simulink model "PIDLoopTest_Multiple"  (R2014a)
settings: Solver=ode3  SolverMode=SingleTasking  StartTime=0.0  StopTime=inf  RelTol=1e-3
libraries: arduinolib x13, simulink x12
settings Model: ExtModeTrigDuration=2  Creator=paddockt  LastModifiedBy=paddockt
settings OptimizationCC: OptimizeModelRefInitCode=on  LifeSpan=1
settings DebuggingCC: UnderspecifiedInitializationDetection=Classic  SolverPrmCheckMsg=none
settings HardwareCC: ProdBitPerInt=16  ProdBitPerPointer=8  ProdIntDivRoundTo=Zero  ProdEndianess=LittleEndian  ProdWordSize=8  ProdHWDeviceType=Atmel->AVR
settings RTWCC: SystemTargetFile=realtime.tlc  GenerateMakefile=off  TemplateMakefile=realtime.tmf  Description=Run on Target Hardware  RTWVerbose=off  ProcessScript=realtime_make_rtw_hook
settings STFCustomTargetCC: TargetLibSuffix=.a  GenerateSampleERTMain=on  ConcurrentExecutionCompliant=off  GeneratePreprocessorConditionals=Use local settings  ERTCustomFileBanners=on  SupportNonInlinedSFcns=off  SupportVariableSizeSignals=on  MATLABClassNameForMDSCustomization=Simulink.SoftwareTarget.ERTCustomization  GRTInterface=off  SystemTargetFile=realtime.tlc
settings ERTTargetCC: CombineOutputUpdateFcns=off  SupportContinuousTime=on  SupportVariableSizeSignals=on  ExtModeMexArgs='192.168.1.20' 1 17725  ERTSrcFileBannerTemplate=realtime_code_template.cgt  ERTHdrFileBannerTemplate=realtime_code_template.cgt  ERTDataSrcFileTemplate=realtime_code_template.cgt  ERTDataHdrFileTemplate=realtime_code_template.cgt  ERTCustomFileTemplate=realtime_file_process.tlc

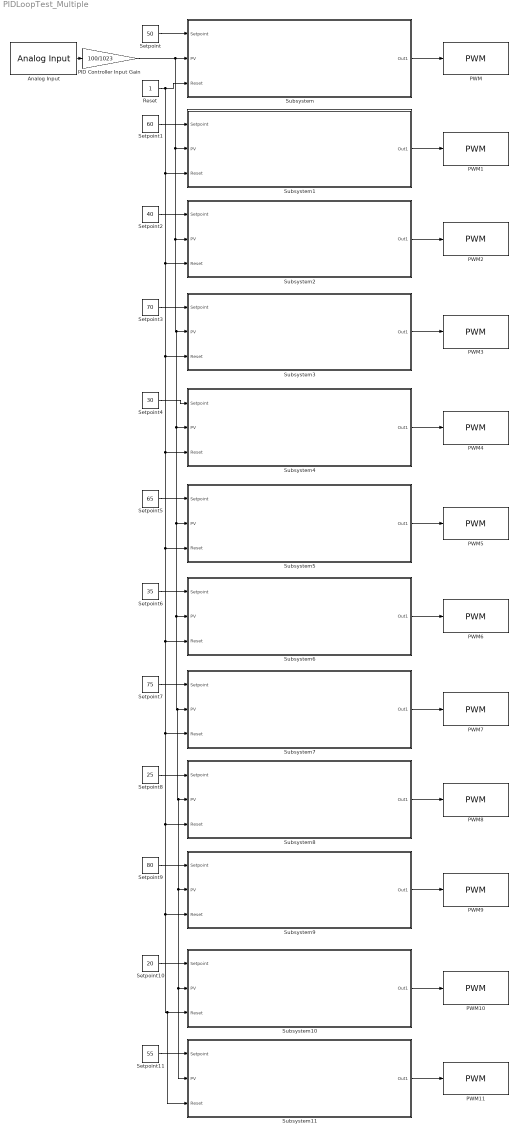
== system PIDLoopTest_Multiple ==
  Analog Input : arduinolib/Analog Input  pinNumber=0  sampleTime=1
  PID Controller Input Gain : Gain  Gain=100/1023
  PWM : arduinolib/PWM  pinNumber=13
  PWM1 : arduinolib/PWM  pinNumber=12
  PWM10 : arduinolib/PWM  pinNumber=3
  PWM11 : arduinolib/PWM  pinNumber=2
  PWM2 : arduinolib/PWM  pinNumber=11
  PWM3 : arduinolib/PWM  pinNumber=10
  PWM4 : arduinolib/PWM  pinNumber=9
  PWM5 : arduinolib/PWM  pinNumber=8
  PWM6 : arduinolib/PWM  pinNumber=7
  PWM7 : arduinolib/PWM  pinNumber=6
  PWM8 : arduinolib/PWM  pinNumber=5
  PWM9 : arduinolib/PWM  pinNumber=4
  Reset : Constant
  Setpoint : Constant  Value=50
  Setpoint1 : Constant  Value=60
  Setpoint10 : Constant  Value=20
  Setpoint11 : Constant  Value=55
  Setpoint2 : Constant  Value=40
  Setpoint3 : Constant  Value=70
  Setpoint4 : Constant  Value=30
  Setpoint5 : Constant  Value=65
  Setpoint6 : Constant  Value=35
  Setpoint7 : Constant  Value=75
  Setpoint8 : Constant  Value=25
  Setpoint9 : Constant  Value=80
  Subsystem : Subsystem
  Subsystem1 : Subsystem
  Subsystem10 : Subsystem
  Subsystem11 : Subsystem
  Subsystem2 : Subsystem
  Subsystem3 : Subsystem
  Subsystem4 : Subsystem
  Subsystem5 : Subsystem
  Subsystem6 : Subsystem
  Subsystem7 : Subsystem
  Subsystem8 : Subsystem
  Subsystem9 : Subsystem
  wires:
  Analog Input/1 -> PID Controller Input Gain/1
  PID Controller Input Gain/1 -> Subsystem11/2(PV), Subsystem10/2(PV), Subsystem9/2(PV), Subsystem8/2(PV), Subsystem7/2(PV), Subsystem6/2(PV), Subsystem5/2(PV), Subsystem4/2(PV), Subsystem3/2(PV), Subsystem2/2(PV), Subsystem1/2(PV), Subsystem/2(PV)
  Setpoint/1 -> Subsystem/1(Setpoint)
  Reset/1 -> Subsystem11/3(Reset), Subsystem10/3(Reset), Subsystem9/3(Reset), Subsystem8/3(Reset), Subsystem7/3(Reset), Subsystem6/3(Reset), Subsystem5/3(Reset), Subsystem4/3(Reset), Subsystem3/3(Reset), Subsystem2/3(Reset), Subsystem1/3(Reset), Subsystem/3(Reset)
  Subsystem/1(Out1) -> PWM/1
  Subsystem1/1(Out1) -> PWM1/1
  Subsystem2/1(Out1) -> PWM2/1
  Subsystem3/1(Out1) -> PWM3/1
  Subsystem4/1(Out1) -> PWM4/1
  Subsystem5/1(Out1) -> PWM5/1
  Subsystem6/1(Out1) -> PWM6/1
  Subsystem7/1(Out1) -> PWM7/1
  Subsystem8/1(Out1) -> PWM8/1
  Subsystem9/1(Out1) -> PWM9/1
  Subsystem10/1(Out1) -> PWM10/1
  Subsystem11/1(Out1) -> PWM11/1
  Setpoint1/1 -> Subsystem1/1(Setpoint)
  Setpoint2/1 -> Subsystem2/1(Setpoint)
  Setpoint3/1 -> Subsystem3/1(Setpoint)
  Setpoint4/1 -> Subsystem4/1(Setpoint)
  Setpoint5/1 -> Subsystem5/1(Setpoint)
  Setpoint6/1 -> Subsystem6/1(Setpoint)
  Setpoint7/1 -> Subsystem7/1(Setpoint)
  Setpoint8/1 -> Subsystem8/1(Setpoint)
  Setpoint9/1 -> Subsystem9/1(Setpoint)
  Setpoint10/1 -> Subsystem10/1(Setpoint)
  Setpoint11/1 -> Subsystem11/1(Setpoint)

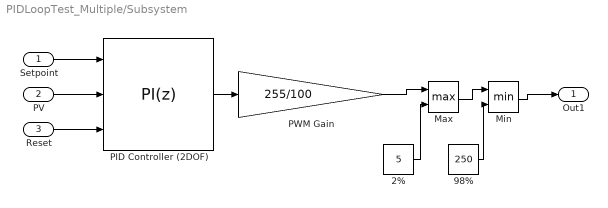
== system PIDLoopTest_Multiple/Subsystem ==
  Setpoint : Inport
  PV : Inport  Port=2
  Reset : Inport  Port=3
  2% : Constant  Value=5
  98% : Constant  Value=250
  Max : MinMax  Function=max  Inputs=2
  Min : MinMax  Inputs=2
  PID Controller (2DOF) : simulink/Continuous/PID Controller (2DOF)  Controller=PI  TimeDomain=Discrete-time  SampleTime=1  IntegratorMethod=Forward Euler  FilterMethod=Forward Euler  Form=Parallel  P=1  I=1  D=0  N=100  b=1  c=1  InitialConditionSource=internal  InitialConditionForIntegrator=0  InitialConditionForFilter=0  ExternalReset=falling  LimitOutput=on  UpperSaturationLimit=100  LowerSaturationLimit=0  LinearizeAsGain=on  AntiWindupMode=none  Kb=1  TrackingMode=off  Kt=1  PParamMin=[]  PParamMax=[]  IParamMin=[]  IParamMax=[]  DParamMin=[]  DParamMax=[]  NParamMin=[]  NParamMax=[]  bParamMin=[]  bParamMax=[]  cParamMin=[]  cParamMax=[]  KbParamMin=[]  KbParamMax=[]  KtParamMin=[]  KtParamMax=[]  POutMin=[]  POutMax=[]  IOutMin=[]  IOutMax=[]  DOutMin=[]  DOutMax=[]  NOutMin=[]  NOutMax=[]  bOutMin=[]  bOutMax=[]  cOutMin=[]  cOutMax=[]  KbOutMin=[]  KbOutMax=[]  KtOutMin=[]  KtOutMax=[]  IntegratorOutMin=[]  IntegratorOutMax=[]  FilterOutMin=[]  FilterOutMax=[]  SumOutMin=[]  SumOutMax=[]  Sum1OutMin=[]  Sum1OutMax=[]  Sum2OutMin=[]  Sum2OutMax=[]  Sum3OutMin=[]  Sum3OutMax=[]  SumI1OutMin=[]  SumI1OutMax=[]  SumI2OutMin=[]  SumI2OutMax=[]  SumI3OutMin=[]  SumI3OutMax=[]  SumDOutMin=[]  SumDOutMax=[]  SaturationOutMin=[]  SaturationOutMax=[]  IntegratorContinuousStateAttributes=''  IntegratorStateMustResolveToSignalObject=off  IntegratorRTWStateStorageClass=Auto  FilterContinuousStateAttributes=''  FilterStateMustResolveToSignalObject=off  FilterRTWStateStorageClass=Auto
  PWM Gain : Gain  Gain=255/100
  Out1 : Outport
  wires:
  PID Controller (2DOF)/1 -> PWM Gain/1
  Setpoint/1 -> PID Controller (2DOF)/1
  PWM Gain/1 -> Max/1
  Reset/1 -> PID Controller (2DOF)/3
  PV/1 -> PID Controller (2DOF)/2
  Min/1 -> Out1/1
  Max/1 -> Min/1
  98%/1 -> Min/2
  2%/1 -> Max/2

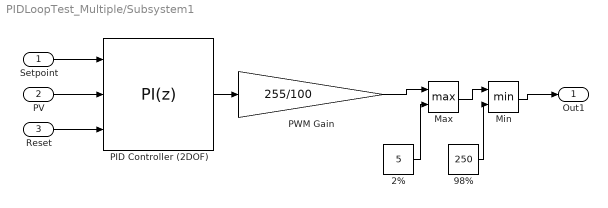
== system PIDLoopTest_Multiple/Subsystem1 ==
  Setpoint : Inport
  PV : Inport  Port=2
  Reset : Inport  Port=3
  2% : Constant  Value=5
  98% : Constant  Value=250
  Max : MinMax  Function=max  Inputs=2
  Min : MinMax  Inputs=2
  PID Controller (2DOF) : simulink/Continuous/PID Controller (2DOF)  Controller=PI  TimeDomain=Discrete-time  SampleTime=1  IntegratorMethod=Forward Euler  FilterMethod=Forward Euler  Form=Parallel  P=1  I=1  D=0  N=100  b=1  c=1  InitialConditionSource=internal  InitialConditionForIntegrator=0  InitialConditionForFilter=0  ExternalReset=falling  LimitOutput=on  UpperSaturationLimit=100  LowerSaturationLimit=0  LinearizeAsGain=on  AntiWindupMode=none  Kb=1  TrackingMode=off  Kt=1  PParamMin=[]  PParamMax=[]  IParamMin=[]  IParamMax=[]  DParamMin=[]  DParamMax=[]  NParamMin=[]  NParamMax=[]  bParamMin=[]  bParamMax=[]  cParamMin=[]  cParamMax=[]  KbParamMin=[]  KbParamMax=[]  KtParamMin=[]  KtParamMax=[]  POutMin=[]  POutMax=[]  IOutMin=[]  IOutMax=[]  DOutMin=[]  DOutMax=[]  NOutMin=[]  NOutMax=[]  bOutMin=[]  bOutMax=[]  cOutMin=[]  cOutMax=[]  KbOutMin=[]  KbOutMax=[]  KtOutMin=[]  KtOutMax=[]  IntegratorOutMin=[]  IntegratorOutMax=[]  FilterOutMin=[]  FilterOutMax=[]  SumOutMin=[]  SumOutMax=[]  Sum1OutMin=[]  Sum1OutMax=[]  Sum2OutMin=[]  Sum2OutMax=[]  Sum3OutMin=[]  Sum3OutMax=[]  SumI1OutMin=[]  SumI1OutMax=[]  SumI2OutMin=[]  SumI2OutMax=[]  SumI3OutMin=[]  SumI3OutMax=[]  SumDOutMin=[]  SumDOutMax=[]  SaturationOutMin=[]  SaturationOutMax=[]  IntegratorContinuousStateAttributes=''  IntegratorStateMustResolveToSignalObject=off  IntegratorRTWStateStorageClass=Auto  FilterContinuousStateAttributes=''  FilterStateMustResolveToSignalObject=off  FilterRTWStateStorageClass=Auto
  PWM Gain : Gain  Gain=255/100
  Out1 : Outport
  wires:
  2%/1 -> Max/2
  98%/1 -> Min/2
  Max/1 -> Min/1
  Min/1 -> Out1/1
  PV/1 -> PID Controller (2DOF)/2
  Reset/1 -> PID Controller (2DOF)/3
  PWM Gain/1 -> Max/1
  Setpoint/1 -> PID Controller (2DOF)/1
  PID Controller (2DOF)/1 -> PWM Gain/1

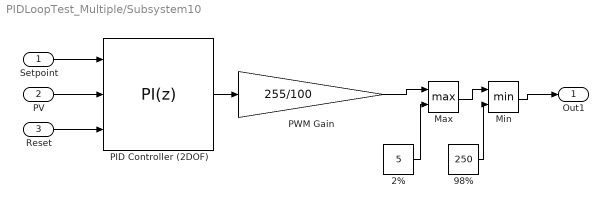
== system PIDLoopTest_Multiple/Subsystem10 ==
  Setpoint : Inport
  PV : Inport  Port=2
  Reset : Inport  Port=3
  2% : Constant  Value=5
  98% : Constant  Value=250
  Max : MinMax  Function=max  Inputs=2
  Min : MinMax  Inputs=2
  PID Controller (2DOF) : simulink/Continuous/PID Controller (2DOF)  Controller=PI  TimeDomain=Discrete-time  SampleTime=1  IntegratorMethod=Forward Euler  FilterMethod=Forward Euler  Form=Parallel  P=1  I=1  D=0  N=100  b=1  c=1  InitialConditionSource=internal  InitialConditionForIntegrator=0  InitialConditionForFilter=0  ExternalReset=falling  LimitOutput=on  UpperSaturationLimit=100  LowerSaturationLimit=0  LinearizeAsGain=on  AntiWindupMode=none  Kb=1  TrackingMode=off  Kt=1  PParamMin=[]  PParamMax=[]  IParamMin=[]  IParamMax=[]  DParamMin=[]  DParamMax=[]  NParamMin=[]  NParamMax=[]  bParamMin=[]  bParamMax=[]  cParamMin=[]  cParamMax=[]  KbParamMin=[]  KbParamMax=[]  KtParamMin=[]  KtParamMax=[]  POutMin=[]  POutMax=[]  IOutMin=[]  IOutMax=[]  DOutMin=[]  DOutMax=[]  NOutMin=[]  NOutMax=[]  bOutMin=[]  bOutMax=[]  cOutMin=[]  cOutMax=[]  KbOutMin=[]  KbOutMax=[]  KtOutMin=[]  KtOutMax=[]  IntegratorOutMin=[]  IntegratorOutMax=[]  FilterOutMin=[]  FilterOutMax=[]  SumOutMin=[]  SumOutMax=[]  Sum1OutMin=[]  Sum1OutMax=[]  Sum2OutMin=[]  Sum2OutMax=[]  Sum3OutMin=[]  Sum3OutMax=[]  SumI1OutMin=[]  SumI1OutMax=[]  SumI2OutMin=[]  SumI2OutMax=[]  SumI3OutMin=[]  SumI3OutMax=[]  SumDOutMin=[]  SumDOutMax=[]  SaturationOutMin=[]  SaturationOutMax=[]  IntegratorContinuousStateAttributes=''  IntegratorStateMustResolveToSignalObject=off  IntegratorRTWStateStorageClass=Auto  FilterContinuousStateAttributes=''  FilterStateMustResolveToSignalObject=off  FilterRTWStateStorageClass=Auto
  PWM Gain : Gain  Gain=255/100
  Out1 : Outport
  wires:
  2%/1 -> Max/2
  98%/1 -> Min/2
  Max/1 -> Min/1
  Min/1 -> Out1/1
  PV/1 -> PID Controller (2DOF)/2
  Reset/1 -> PID Controller (2DOF)/3
  PWM Gain/1 -> Max/1
  Setpoint/1 -> PID Controller (2DOF)/1
  PID Controller (2DOF)/1 -> PWM Gain/1

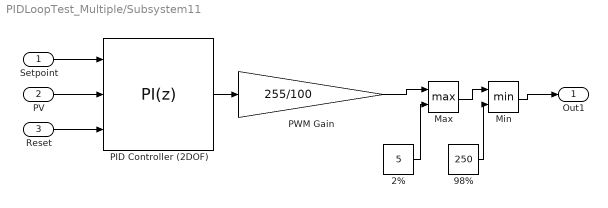
== system PIDLoopTest_Multiple/Subsystem11 ==
  Setpoint : Inport
  PV : Inport  Port=2
  Reset : Inport  Port=3
  2% : Constant  Value=5
  98% : Constant  Value=250
  Max : MinMax  Function=max  Inputs=2
  Min : MinMax  Inputs=2
  PID Controller (2DOF) : simulink/Continuous/PID Controller (2DOF)  Controller=PI  TimeDomain=Discrete-time  SampleTime=1  IntegratorMethod=Forward Euler  FilterMethod=Forward Euler  Form=Parallel  P=1  I=1  D=0  N=100  b=1  c=1  InitialConditionSource=internal  InitialConditionForIntegrator=0  InitialConditionForFilter=0  ExternalReset=falling  LimitOutput=on  UpperSaturationLimit=100  LowerSaturationLimit=0  LinearizeAsGain=on  AntiWindupMode=none  Kb=1  TrackingMode=off  Kt=1  PParamMin=[]  PParamMax=[]  IParamMin=[]  IParamMax=[]  DParamMin=[]  DParamMax=[]  NParamMin=[]  NParamMax=[]  bParamMin=[]  bParamMax=[]  cParamMin=[]  cParamMax=[]  KbParamMin=[]  KbParamMax=[]  KtParamMin=[]  KtParamMax=[]  POutMin=[]  POutMax=[]  IOutMin=[]  IOutMax=[]  DOutMin=[]  DOutMax=[]  NOutMin=[]  NOutMax=[]  bOutMin=[]  bOutMax=[]  cOutMin=[]  cOutMax=[]  KbOutMin=[]  KbOutMax=[]  KtOutMin=[]  KtOutMax=[]  IntegratorOutMin=[]  IntegratorOutMax=[]  FilterOutMin=[]  FilterOutMax=[]  SumOutMin=[]  SumOutMax=[]  Sum1OutMin=[]  Sum1OutMax=[]  Sum2OutMin=[]  Sum2OutMax=[]  Sum3OutMin=[]  Sum3OutMax=[]  SumI1OutMin=[]  SumI1OutMax=[]  SumI2OutMin=[]  SumI2OutMax=[]  SumI3OutMin=[]  SumI3OutMax=[]  SumDOutMin=[]  SumDOutMax=[]  SaturationOutMin=[]  SaturationOutMax=[]  IntegratorContinuousStateAttributes=''  IntegratorStateMustResolveToSignalObject=off  IntegratorRTWStateStorageClass=Auto  FilterContinuousStateAttributes=''  FilterStateMustResolveToSignalObject=off  FilterRTWStateStorageClass=Auto
  PWM Gain : Gain  Gain=255/100
  Out1 : Outport
  wires:
  PID Controller (2DOF)/1 -> PWM Gain/1
  Setpoint/1 -> PID Controller (2DOF)/1
  PWM Gain/1 -> Max/1
  Reset/1 -> PID Controller (2DOF)/3
  PV/1 -> PID Controller (2DOF)/2
  Min/1 -> Out1/1
  Max/1 -> Min/1
  98%/1 -> Min/2
  2%/1 -> Max/2

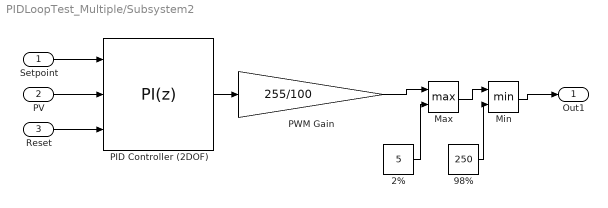
== system PIDLoopTest_Multiple/Subsystem2 ==
  Setpoint : Inport
  PV : Inport  Port=2
  Reset : Inport  Port=3
  2% : Constant  Value=5
  98% : Constant  Value=250
  Max : MinMax  Function=max  Inputs=2
  Min : MinMax  Inputs=2
  PID Controller (2DOF) : simulink/Continuous/PID Controller (2DOF)  Controller=PI  TimeDomain=Discrete-time  SampleTime=1  IntegratorMethod=Forward Euler  FilterMethod=Forward Euler  Form=Parallel  P=1  I=1  D=0  N=100  b=1  c=1  InitialConditionSource=internal  InitialConditionForIntegrator=0  InitialConditionForFilter=0  ExternalReset=falling  LimitOutput=on  UpperSaturationLimit=100  LowerSaturationLimit=0  LinearizeAsGain=on  AntiWindupMode=none  Kb=1  TrackingMode=off  Kt=1  PParamMin=[]  PParamMax=[]  IParamMin=[]  IParamMax=[]  DParamMin=[]  DParamMax=[]  NParamMin=[]  NParamMax=[]  bParamMin=[]  bParamMax=[]  cParamMin=[]  cParamMax=[]  KbParamMin=[]  KbParamMax=[]  KtParamMin=[]  KtParamMax=[]  POutMin=[]  POutMax=[]  IOutMin=[]  IOutMax=[]  DOutMin=[]  DOutMax=[]  NOutMin=[]  NOutMax=[]  bOutMin=[]  bOutMax=[]  cOutMin=[]  cOutMax=[]  KbOutMin=[]  KbOutMax=[]  KtOutMin=[]  KtOutMax=[]  IntegratorOutMin=[]  IntegratorOutMax=[]  FilterOutMin=[]  FilterOutMax=[]  SumOutMin=[]  SumOutMax=[]  Sum1OutMin=[]  Sum1OutMax=[]  Sum2OutMin=[]  Sum2OutMax=[]  Sum3OutMin=[]  Sum3OutMax=[]  SumI1OutMin=[]  SumI1OutMax=[]  SumI2OutMin=[]  SumI2OutMax=[]  SumI3OutMin=[]  SumI3OutMax=[]  SumDOutMin=[]  SumDOutMax=[]  SaturationOutMin=[]  SaturationOutMax=[]  IntegratorContinuousStateAttributes=''  IntegratorStateMustResolveToSignalObject=off  IntegratorRTWStateStorageClass=Auto  FilterContinuousStateAttributes=''  FilterStateMustResolveToSignalObject=off  FilterRTWStateStorageClass=Auto
  PWM Gain : Gain  Gain=255/100
  Out1 : Outport
  wires:
  2%/1 -> Max/2
  98%/1 -> Min/2
  Max/1 -> Min/1
  Min/1 -> Out1/1
  PV/1 -> PID Controller (2DOF)/2
  Reset/1 -> PID Controller (2DOF)/3
  PWM Gain/1 -> Max/1
  Setpoint/1 -> PID Controller (2DOF)/1
  PID Controller (2DOF)/1 -> PWM Gain/1

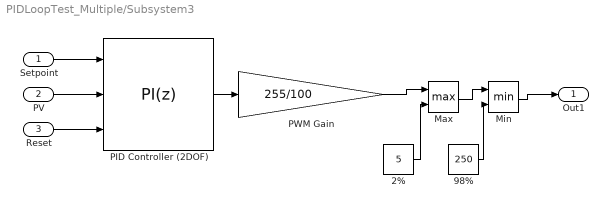
== system PIDLoopTest_Multiple/Subsystem3 ==
  Setpoint : Inport
  PV : Inport  Port=2
  Reset : Inport  Port=3
  2% : Constant  Value=5
  98% : Constant  Value=250
  Max : MinMax  Function=max  Inputs=2
  Min : MinMax  Inputs=2
  PID Controller (2DOF) : simulink/Continuous/PID Controller (2DOF)  Controller=PI  TimeDomain=Discrete-time  SampleTime=1  IntegratorMethod=Forward Euler  FilterMethod=Forward Euler  Form=Parallel  P=1  I=1  D=0  N=100  b=1  c=1  InitialConditionSource=internal  InitialConditionForIntegrator=0  InitialConditionForFilter=0  ExternalReset=falling  LimitOutput=on  UpperSaturationLimit=100  LowerSaturationLimit=0  LinearizeAsGain=on  AntiWindupMode=none  Kb=1  TrackingMode=off  Kt=1  PParamMin=[]  PParamMax=[]  IParamMin=[]  IParamMax=[]  DParamMin=[]  DParamMax=[]  NParamMin=[]  NParamMax=[]  bParamMin=[]  bParamMax=[]  cParamMin=[]  cParamMax=[]  KbParamMin=[]  KbParamMax=[]  KtParamMin=[]  KtParamMax=[]  POutMin=[]  POutMax=[]  IOutMin=[]  IOutMax=[]  DOutMin=[]  DOutMax=[]  NOutMin=[]  NOutMax=[]  bOutMin=[]  bOutMax=[]  cOutMin=[]  cOutMax=[]  KbOutMin=[]  KbOutMax=[]  KtOutMin=[]  KtOutMax=[]  IntegratorOutMin=[]  IntegratorOutMax=[]  FilterOutMin=[]  FilterOutMax=[]  SumOutMin=[]  SumOutMax=[]  Sum1OutMin=[]  Sum1OutMax=[]  Sum2OutMin=[]  Sum2OutMax=[]  Sum3OutMin=[]  Sum3OutMax=[]  SumI1OutMin=[]  SumI1OutMax=[]  SumI2OutMin=[]  SumI2OutMax=[]  SumI3OutMin=[]  SumI3OutMax=[]  SumDOutMin=[]  SumDOutMax=[]  SaturationOutMin=[]  SaturationOutMax=[]  IntegratorContinuousStateAttributes=''  IntegratorStateMustResolveToSignalObject=off  IntegratorRTWStateStorageClass=Auto  FilterContinuousStateAttributes=''  FilterStateMustResolveToSignalObject=off  FilterRTWStateStorageClass=Auto
  PWM Gain : Gain  Gain=255/100
  Out1 : Outport
  wires:
  PID Controller (2DOF)/1 -> PWM Gain/1
  Setpoint/1 -> PID Controller (2DOF)/1
  PWM Gain/1 -> Max/1
  Reset/1 -> PID Controller (2DOF)/3
  PV/1 -> PID Controller (2DOF)/2
  Min/1 -> Out1/1
  Max/1 -> Min/1
  98%/1 -> Min/2
  2%/1 -> Max/2

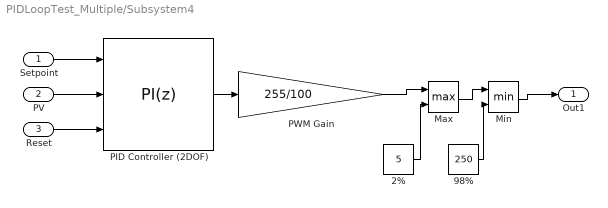
== system PIDLoopTest_Multiple/Subsystem4 ==
  Setpoint : Inport
  PV : Inport  Port=2
  Reset : Inport  Port=3
  2% : Constant  Value=5
  98% : Constant  Value=250
  Max : MinMax  Function=max  Inputs=2
  Min : MinMax  Inputs=2
  PID Controller (2DOF) : simulink/Continuous/PID Controller (2DOF)  Controller=PI  TimeDomain=Discrete-time  SampleTime=1  IntegratorMethod=Forward Euler  FilterMethod=Forward Euler  Form=Parallel  P=1  I=1  D=0  N=100  b=1  c=1  InitialConditionSource=internal  InitialConditionForIntegrator=0  InitialConditionForFilter=0  ExternalReset=falling  LimitOutput=on  UpperSaturationLimit=100  LowerSaturationLimit=0  LinearizeAsGain=on  AntiWindupMode=none  Kb=1  TrackingMode=off  Kt=1  PParamMin=[]  PParamMax=[]  IParamMin=[]  IParamMax=[]  DParamMin=[]  DParamMax=[]  NParamMin=[]  NParamMax=[]  bParamMin=[]  bParamMax=[]  cParamMin=[]  cParamMax=[]  KbParamMin=[]  KbParamMax=[]  KtParamMin=[]  KtParamMax=[]  POutMin=[]  POutMax=[]  IOutMin=[]  IOutMax=[]  DOutMin=[]  DOutMax=[]  NOutMin=[]  NOutMax=[]  bOutMin=[]  bOutMax=[]  cOutMin=[]  cOutMax=[]  KbOutMin=[]  KbOutMax=[]  KtOutMin=[]  KtOutMax=[]  IntegratorOutMin=[]  IntegratorOutMax=[]  FilterOutMin=[]  FilterOutMax=[]  SumOutMin=[]  SumOutMax=[]  Sum1OutMin=[]  Sum1OutMax=[]  Sum2OutMin=[]  Sum2OutMax=[]  Sum3OutMin=[]  Sum3OutMax=[]  SumI1OutMin=[]  SumI1OutMax=[]  SumI2OutMin=[]  SumI2OutMax=[]  SumI3OutMin=[]  SumI3OutMax=[]  SumDOutMin=[]  SumDOutMax=[]  SaturationOutMin=[]  SaturationOutMax=[]  IntegratorContinuousStateAttributes=''  IntegratorStateMustResolveToSignalObject=off  IntegratorRTWStateStorageClass=Auto  FilterContinuousStateAttributes=''  FilterStateMustResolveToSignalObject=off  FilterRTWStateStorageClass=Auto
  PWM Gain : Gain  Gain=255/100
  Out1 : Outport
  wires:
  2%/1 -> Max/2
  98%/1 -> Min/2
  Max/1 -> Min/1
  Min/1 -> Out1/1
  PV/1 -> PID Controller (2DOF)/2
  Reset/1 -> PID Controller (2DOF)/3
  PWM Gain/1 -> Max/1
  Setpoint/1 -> PID Controller (2DOF)/1
  PID Controller (2DOF)/1 -> PWM Gain/1

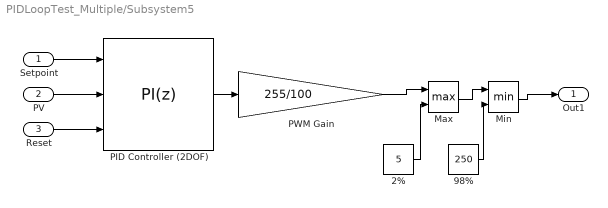
== system PIDLoopTest_Multiple/Subsystem5 ==
  Setpoint : Inport
  PV : Inport  Port=2
  Reset : Inport  Port=3
  2% : Constant  Value=5
  98% : Constant  Value=250
  Max : MinMax  Function=max  Inputs=2
  Min : MinMax  Inputs=2
  PID Controller (2DOF) : simulink/Continuous/PID Controller (2DOF)  Controller=PI  TimeDomain=Discrete-time  SampleTime=1  IntegratorMethod=Forward Euler  FilterMethod=Forward Euler  Form=Parallel  P=1  I=1  D=0  N=100  b=1  c=1  InitialConditionSource=internal  InitialConditionForIntegrator=0  InitialConditionForFilter=0  ExternalReset=falling  LimitOutput=on  UpperSaturationLimit=100  LowerSaturationLimit=0  LinearizeAsGain=on  AntiWindupMode=none  Kb=1  TrackingMode=off  Kt=1  PParamMin=[]  PParamMax=[]  IParamMin=[]  IParamMax=[]  DParamMin=[]  DParamMax=[]  NParamMin=[]  NParamMax=[]  bParamMin=[]  bParamMax=[]  cParamMin=[]  cParamMax=[]  KbParamMin=[]  KbParamMax=[]  KtParamMin=[]  KtParamMax=[]  POutMin=[]  POutMax=[]  IOutMin=[]  IOutMax=[]  DOutMin=[]  DOutMax=[]  NOutMin=[]  NOutMax=[]  bOutMin=[]  bOutMax=[]  cOutMin=[]  cOutMax=[]  KbOutMin=[]  KbOutMax=[]  KtOutMin=[]  KtOutMax=[]  IntegratorOutMin=[]  IntegratorOutMax=[]  FilterOutMin=[]  FilterOutMax=[]  SumOutMin=[]  SumOutMax=[]  Sum1OutMin=[]  Sum1OutMax=[]  Sum2OutMin=[]  Sum2OutMax=[]  Sum3OutMin=[]  Sum3OutMax=[]  SumI1OutMin=[]  SumI1OutMax=[]  SumI2OutMin=[]  SumI2OutMax=[]  SumI3OutMin=[]  SumI3OutMax=[]  SumDOutMin=[]  SumDOutMax=[]  SaturationOutMin=[]  SaturationOutMax=[]  IntegratorContinuousStateAttributes=''  IntegratorStateMustResolveToSignalObject=off  IntegratorRTWStateStorageClass=Auto  FilterContinuousStateAttributes=''  FilterStateMustResolveToSignalObject=off  FilterRTWStateStorageClass=Auto
  PWM Gain : Gain  Gain=255/100
  Out1 : Outport
  wires:
  PID Controller (2DOF)/1 -> PWM Gain/1
  Setpoint/1 -> PID Controller (2DOF)/1
  PWM Gain/1 -> Max/1
  Reset/1 -> PID Controller (2DOF)/3
  PV/1 -> PID Controller (2DOF)/2
  Min/1 -> Out1/1
  Max/1 -> Min/1
  98%/1 -> Min/2
  2%/1 -> Max/2

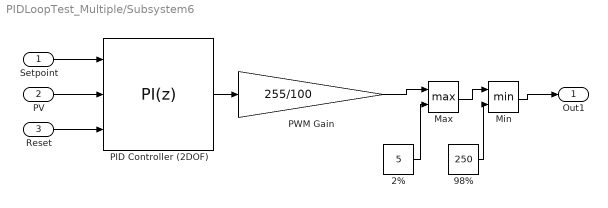
== system PIDLoopTest_Multiple/Subsystem6 ==
  Setpoint : Inport
  PV : Inport  Port=2
  Reset : Inport  Port=3
  2% : Constant  Value=5
  98% : Constant  Value=250
  Max : MinMax  Function=max  Inputs=2
  Min : MinMax  Inputs=2
  PID Controller (2DOF) : simulink/Continuous/PID Controller (2DOF)  Controller=PI  TimeDomain=Discrete-time  SampleTime=1  IntegratorMethod=Forward Euler  FilterMethod=Forward Euler  Form=Parallel  P=1  I=1  D=0  N=100  b=1  c=1  InitialConditionSource=internal  InitialConditionForIntegrator=0  InitialConditionForFilter=0  ExternalReset=falling  LimitOutput=on  UpperSaturationLimit=100  LowerSaturationLimit=0  LinearizeAsGain=on  AntiWindupMode=none  Kb=1  TrackingMode=off  Kt=1  PParamMin=[]  PParamMax=[]  IParamMin=[]  IParamMax=[]  DParamMin=[]  DParamMax=[]  NParamMin=[]  NParamMax=[]  bParamMin=[]  bParamMax=[]  cParamMin=[]  cParamMax=[]  KbParamMin=[]  KbParamMax=[]  KtParamMin=[]  KtParamMax=[]  POutMin=[]  POutMax=[]  IOutMin=[]  IOutMax=[]  DOutMin=[]  DOutMax=[]  NOutMin=[]  NOutMax=[]  bOutMin=[]  bOutMax=[]  cOutMin=[]  cOutMax=[]  KbOutMin=[]  KbOutMax=[]  KtOutMin=[]  KtOutMax=[]  IntegratorOutMin=[]  IntegratorOutMax=[]  FilterOutMin=[]  FilterOutMax=[]  SumOutMin=[]  SumOutMax=[]  Sum1OutMin=[]  Sum1OutMax=[]  Sum2OutMin=[]  Sum2OutMax=[]  Sum3OutMin=[]  Sum3OutMax=[]  SumI1OutMin=[]  SumI1OutMax=[]  SumI2OutMin=[]  SumI2OutMax=[]  SumI3OutMin=[]  SumI3OutMax=[]  SumDOutMin=[]  SumDOutMax=[]  SaturationOutMin=[]  SaturationOutMax=[]  IntegratorContinuousStateAttributes=''  IntegratorStateMustResolveToSignalObject=off  IntegratorRTWStateStorageClass=Auto  FilterContinuousStateAttributes=''  FilterStateMustResolveToSignalObject=off  FilterRTWStateStorageClass=Auto
  PWM Gain : Gain  Gain=255/100
  Out1 : Outport
  wires:
  PID Controller (2DOF)/1 -> PWM Gain/1
  Setpoint/1 -> PID Controller (2DOF)/1
  PWM Gain/1 -> Max/1
  Reset/1 -> PID Controller (2DOF)/3
  PV/1 -> PID Controller (2DOF)/2
  Min/1 -> Out1/1
  Max/1 -> Min/1
  98%/1 -> Min/2
  2%/1 -> Max/2

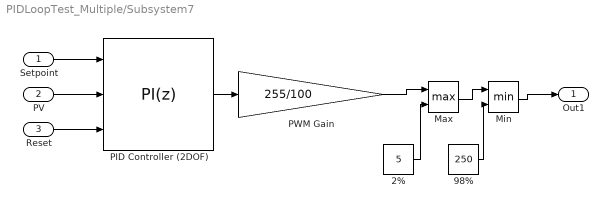
== system PIDLoopTest_Multiple/Subsystem7 ==
  Setpoint : Inport
  PV : Inport  Port=2
  Reset : Inport  Port=3
  2% : Constant  Value=5
  98% : Constant  Value=250
  Max : MinMax  Function=max  Inputs=2
  Min : MinMax  Inputs=2
  PID Controller (2DOF) : simulink/Continuous/PID Controller (2DOF)  Controller=PI  TimeDomain=Discrete-time  SampleTime=1  IntegratorMethod=Forward Euler  FilterMethod=Forward Euler  Form=Parallel  P=1  I=1  D=0  N=100  b=1  c=1  InitialConditionSource=internal  InitialConditionForIntegrator=0  InitialConditionForFilter=0  ExternalReset=falling  LimitOutput=on  UpperSaturationLimit=100  LowerSaturationLimit=0  LinearizeAsGain=on  AntiWindupMode=none  Kb=1  TrackingMode=off  Kt=1  PParamMin=[]  PParamMax=[]  IParamMin=[]  IParamMax=[]  DParamMin=[]  DParamMax=[]  NParamMin=[]  NParamMax=[]  bParamMin=[]  bParamMax=[]  cParamMin=[]  cParamMax=[]  KbParamMin=[]  KbParamMax=[]  KtParamMin=[]  KtParamMax=[]  POutMin=[]  POutMax=[]  IOutMin=[]  IOutMax=[]  DOutMin=[]  DOutMax=[]  NOutMin=[]  NOutMax=[]  bOutMin=[]  bOutMax=[]  cOutMin=[]  cOutMax=[]  KbOutMin=[]  KbOutMax=[]  KtOutMin=[]  KtOutMax=[]  IntegratorOutMin=[]  IntegratorOutMax=[]  FilterOutMin=[]  FilterOutMax=[]  SumOutMin=[]  SumOutMax=[]  Sum1OutMin=[]  Sum1OutMax=[]  Sum2OutMin=[]  Sum2OutMax=[]  Sum3OutMin=[]  Sum3OutMax=[]  SumI1OutMin=[]  SumI1OutMax=[]  SumI2OutMin=[]  SumI2OutMax=[]  SumI3OutMin=[]  SumI3OutMax=[]  SumDOutMin=[]  SumDOutMax=[]  SaturationOutMin=[]  SaturationOutMax=[]  IntegratorContinuousStateAttributes=''  IntegratorStateMustResolveToSignalObject=off  IntegratorRTWStateStorageClass=Auto  FilterContinuousStateAttributes=''  FilterStateMustResolveToSignalObject=off  FilterRTWStateStorageClass=Auto
  PWM Gain : Gain  Gain=255/100
  Out1 : Outport
  wires:
  2%/1 -> Max/2
  98%/1 -> Min/2
  Max/1 -> Min/1
  Min/1 -> Out1/1
  PV/1 -> PID Controller (2DOF)/2
  Reset/1 -> PID Controller (2DOF)/3
  PWM Gain/1 -> Max/1
  Setpoint/1 -> PID Controller (2DOF)/1
  PID Controller (2DOF)/1 -> PWM Gain/1

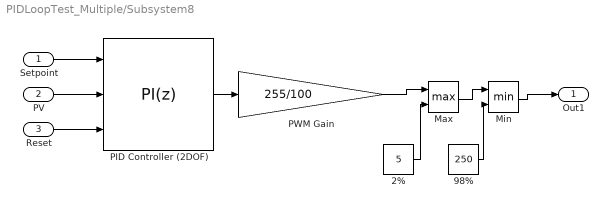
== system PIDLoopTest_Multiple/Subsystem8 ==
  Setpoint : Inport
  PV : Inport  Port=2
  Reset : Inport  Port=3
  2% : Constant  Value=5
  98% : Constant  Value=250
  Max : MinMax  Function=max  Inputs=2
  Min : MinMax  Inputs=2
  PID Controller (2DOF) : simulink/Continuous/PID Controller (2DOF)  Controller=PI  TimeDomain=Discrete-time  SampleTime=1  IntegratorMethod=Forward Euler  FilterMethod=Forward Euler  Form=Parallel  P=1  I=1  D=0  N=100  b=1  c=1  InitialConditionSource=internal  InitialConditionForIntegrator=0  InitialConditionForFilter=0  ExternalReset=falling  LimitOutput=on  UpperSaturationLimit=100  LowerSaturationLimit=0  LinearizeAsGain=on  AntiWindupMode=none  Kb=1  TrackingMode=off  Kt=1  PParamMin=[]  PParamMax=[]  IParamMin=[]  IParamMax=[]  DParamMin=[]  DParamMax=[]  NParamMin=[]  NParamMax=[]  bParamMin=[]  bParamMax=[]  cParamMin=[]  cParamMax=[]  KbParamMin=[]  KbParamMax=[]  KtParamMin=[]  KtParamMax=[]  POutMin=[]  POutMax=[]  IOutMin=[]  IOutMax=[]  DOutMin=[]  DOutMax=[]  NOutMin=[]  NOutMax=[]  bOutMin=[]  bOutMax=[]  cOutMin=[]  cOutMax=[]  KbOutMin=[]  KbOutMax=[]  KtOutMin=[]  KtOutMax=[]  IntegratorOutMin=[]  IntegratorOutMax=[]  FilterOutMin=[]  FilterOutMax=[]  SumOutMin=[]  SumOutMax=[]  Sum1OutMin=[]  Sum1OutMax=[]  Sum2OutMin=[]  Sum2OutMax=[]  Sum3OutMin=[]  Sum3OutMax=[]  SumI1OutMin=[]  SumI1OutMax=[]  SumI2OutMin=[]  SumI2OutMax=[]  SumI3OutMin=[]  SumI3OutMax=[]  SumDOutMin=[]  SumDOutMax=[]  SaturationOutMin=[]  SaturationOutMax=[]  IntegratorContinuousStateAttributes=''  IntegratorStateMustResolveToSignalObject=off  IntegratorRTWStateStorageClass=Auto  FilterContinuousStateAttributes=''  FilterStateMustResolveToSignalObject=off  FilterRTWStateStorageClass=Auto
  PWM Gain : Gain  Gain=255/100
  Out1 : Outport
  wires:
  PID Controller (2DOF)/1 -> PWM Gain/1
  Setpoint/1 -> PID Controller (2DOF)/1
  PWM Gain/1 -> Max/1
  Reset/1 -> PID Controller (2DOF)/3
  PV/1 -> PID Controller (2DOF)/2
  Min/1 -> Out1/1
  Max/1 -> Min/1
  98%/1 -> Min/2
  2%/1 -> Max/2

== system PIDLoopTest_Multiple/Subsystem9 ==
  Setpoint : Inport
  PV : Inport  Port=2
  Reset : Inport  Port=3
  2% : Constant  Value=5
  98% : Constant  Value=250
  Max : MinMax  Function=max  Inputs=2
  Min : MinMax  Inputs=2
  PID Controller (2DOF) : simulink/Continuous/PID Controller (2DOF)  Controller=PI  TimeDomain=Discrete-time  SampleTime=1  IntegratorMethod=Forward Euler  FilterMethod=Forward Euler  Form=Parallel  P=1  I=1  D=0  N=100  b=1  c=1  InitialConditionSource=internal  InitialConditionForIntegrator=0  InitialConditionForFilter=0  ExternalReset=falling  LimitOutput=on  UpperSaturationLimit=100  LowerSaturationLimit=0  LinearizeAsGain=on  AntiWindupMode=none  Kb=1  TrackingMode=off  Kt=1  PParamMin=[]  PParamMax=[]  IParamMin=[]  IParamMax=[]  DParamMin=[]  DParamMax=[]  NParamMin=[]  NParamMax=[]  bParamMin=[]  bParamMax=[]  cParamMin=[]  cParamMax=[]  KbParamMin=[]  KbParamMax=[]  KtParamMin=[]  KtParamMax=[]  POutMin=[]  POutMax=[]  IOutMin=[]  IOutMax=[]  DOutMin=[]  DOutMax=[]  NOutMin=[]  NOutMax=[]  bOutMin=[]  bOutMax=[]  cOutMin=[]  cOutMax=[]  KbOutMin=[]  KbOutMax=[]  KtOutMin=[]  KtOutMax=[]  IntegratorOutMin=[]  IntegratorOutMax=[]  FilterOutMin=[]  FilterOutMax=[]  SumOutMin=[]  SumOutMax=[]  Sum1OutMin=[]  Sum1OutMax=[]  Sum2OutMin=[]  Sum2OutMax=[]  Sum3OutMin=[]  Sum3OutMax=[]  SumI1OutMin=[]  SumI1OutMax=[]  SumI2OutMin=[]  SumI2OutMax=[]  SumI3OutMin=[]  SumI3OutMax=[]  SumDOutMin=[]  SumDOutMax=[]  SaturationOutMin=[]  SaturationOutMax=[]  IntegratorContinuousStateAttributes=''  IntegratorStateMustResolveToSignalObject=off  IntegratorRTWStateStorageClass=Auto  FilterContinuousStateAttributes=''  FilterStateMustResolveToSignalObject=off  FilterRTWStateStorageClass=Auto
  PWM Gain : Gain  Gain=255/100
  Out1 : Outport
  wires:
  2%/1 -> Max/2
  98%/1 -> Min/2
  Max/1 -> Min/1
  Min/1 -> Out1/1
  PV/1 -> PID Controller (2DOF)/2
  Reset/1 -> PID Controller (2DOF)/3
  PWM Gain/1 -> Max/1
  Setpoint/1 -> PID Controller (2DOF)/1
  PID Controller (2DOF)/1 -> PWM Gain/1
